simulink model "F550_Openloop"  (R2024a)
settings: Solver=VariableStepAuto  StartTime=0.0  StopTime=100  FixedStep=0.001  RelTol=1e-3
undefined symbols (not defined in the file): r2d
settings Model: Creator=ADMIN  LastModifiedBy=CNU_UASG
settings DataIOCC: ExternalInput=getinputstruct(op_trim1)  InitialState=getstatestruct(op_trim1)
settings DebuggingCC: UnconnectedInputMsg=warning  UnconnectedOutputMsg=warning  UnconnectedLineMsg=warning
settings ModelReferenceCC: EnableRefExpFcnMdlSchedulingChecks=on
settings RTWCC: GPUComputeCapability=3.5  DLArmComputeVersion=19.05

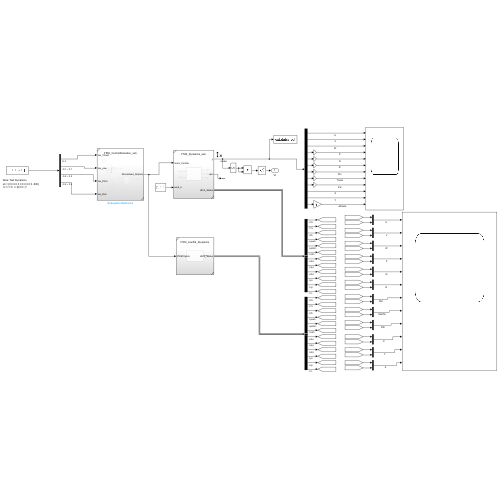
[thumbnail: Simulink's stored preview of the top-level diagram]
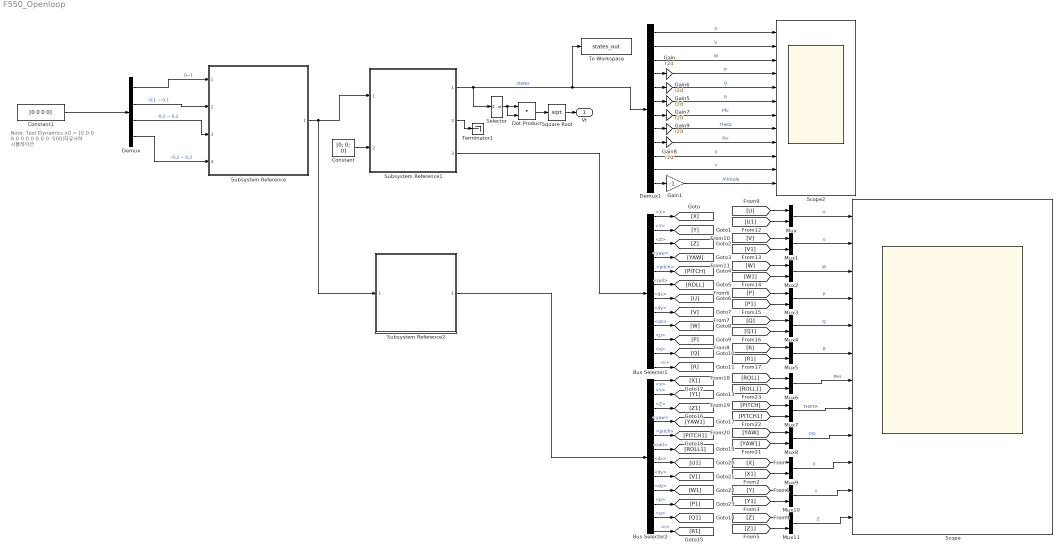
== system F550_Openloop ==
  note: Note: Test Dynamics
      | x0 = [0 0 0 0 0 0 0 0 0 0 0 -500]
      | 자유낙하 시뮬레이션
  Bus Selector1 : BusSelector  OutputSignals=X,Y,Z,yaw,pitch,roll,dx,dy,dz,p,q,r
  Bus Selector2 : BusSelector  OutputSignals=X,Y,Z,yaw,pitch,roll,dx,dy,dz,p,q,r
  Constant : Constant  Value=[0; 0; 0]
  Constant1 : Constant  Value=[0 0 0 0]
  Demux : Demux
  Demux1 : Demux  Outputs=12
  Dot Product : DotProduct  OutDataTypeStr=Inherit: Inherit via internal rule
  Gain{,5..9} (6 alike) : Gain  Gain=r2d
  Gain1 : Gain  Gain=-1
  Mux{,1..11} (12 alike) : Mux  Inputs=2
  Scope : Scope  NumInputPorts=12
  Scope2 : Scope  NumInputPorts=12
  Selector : Selector  InputPortWidth=12  IndexOptions=Index vector (dialog)  Indices=[1 2 3]  OutputSizes=1
  Square Root : Sqrt
  Subsystem Reference : Subsystem  ReferencedSubsystem=F550_ControlAllocation_sub
  Subsystem Reference1 : Subsystem  ReferencedSubsystem=F550_Dynamics_sub
  Subsystem Reference2 : Subsystem  ReferencedSubsystem=F550_LowFid_Dynamics
  Terminator1 : Terminator
  To Workspace : ToWorkspace  VariableName=states_out  SampleTime=-1
  Vt : Outport
  wires:
  Demux/4 -> Subsystem Reference/4  "-0.2 ~ 0.2"
  Demux/3 -> Subsystem Reference/3  "-0.2 ~ 0.2"
  Demux/2 -> Subsystem Reference/2  "-0.1 ~ 0.1"
  Demux/1 -> Subsystem Reference/1  "0~1"
  Selector/1 -> Dot Product/1, Dot Product/2
  Square Root/1 -> Vt/1
  Dot Product/1 -> Square Root/1
  Subsystem Reference1/1 -> Demux1/1, To Workspace/1, Selector/1  "states"
  Subsystem Reference1/3 -> Bus Selector1/1
  Constant/1 -> Subsystem Reference1/2
  Subsystem Reference/1 -> Subsystem Reference2/1, Subsystem Reference1/1
  Subsystem Reference1/2 -> Terminator1/1
  Gain5/1 -> Scope2/6  "R"
  Demux1/9 -> Gain8/1
  Demux1/7 -> Gain7/1
  Demux1/3 -> Scope2/3  "W"
  Demux1/1 -> Scope2/1  "U"
  Demux1/2 -> Scope2/2  "V"
  Demux1/4 -> Gain/1
  Gain8/1 -> Scope2/9  "Psi"
  Gain7/1 -> Scope2/7  "Phi"
  Demux1/8 -> Gain9/1
  Demux1/5 -> Gain6/1
  Gain/1 -> Scope2/4  "P"
  Gain6/1 -> Scope2/5  "Q"
  Gain9/1 -> Scope2/8  "Theta"
  Demux1/6 -> Gain5/1
  Demux1/10 -> Scope2/10  "X"
  Demux1/11 -> Scope2/11  "Y"
  Demux1/12 -> Gain1/1
  Gain1/1 -> Scope2/12  "Altitude"
  Constant1/1 -> Demux/1
  Subsystem Reference2/1 -> Bus Selector2/1
  [Y1] -> Mux10/2
  [V1] -> Mux1/2
  Mux7/1 -> Scope/8  "THETA"
  Bus Selector2/7 -> [U1]  "<dx>"
  [U] -> Mux/1
  Mux9/1 -> Scope/10  "X"
  Bus Selector1/1 -> [X]  "<X>"
  [Y] -> Mux10/1
  [X] -> Mux9/1
  [Z] -> Mux11/1
  [R1] -> Mux5/2
  Mux8/1 -> Scope/9  "PSI"
  Mux6/1 -> Scope/7  "PHI"
  Mux5/1 -> Scope/6  "R"
  Mux4/1 -> Scope/5  "Q"
  Mux1/1 -> Scope/2  "V"
  Bus Selector2/12 -> [R1]  "<r>"
  [W] -> Mux2/1
  [PITCH] -> Mux7/1
  [W1] -> Mux2/2
  Bus Selector1/11 -> [Q]  "<q>"
  [Z1] -> Mux11/2
  [R] -> Mux5/1
  Bus Selector2/3 -> [Z1]  "<Z>"
  [Q1] -> Mux4/2
  [YAW1] -> Mux8/2
  [P] -> Mux3/1
  [PITCH1] -> Mux7/2
  [V] -> Mux1/1
  [U1] -> Mux/2
  [P1] -> Mux3/2
  [Q] -> Mux4/1
  Bus Selector1/10 -> [P]  "<p>"
  Bus Selector2/10 -> [P1]  "<p>"
  [ROLL1] -> Mux6/2
  Mux10/1 -> Scope/11  "Y"
  [ROLL] -> Mux6/1
  Mux/1 -> Scope/1  "U"
  Bus Selector2/11 -> [Q1]  "<q>"
  Bus Selector2/4 -> [YAW1]  "<yaw>"
  Bus Selector1/12 -> [R]  "<r>"
  Bus Selector2/9 -> [W1]  "<dz>"
  [X1] -> Mux9/2
  Bus Selector2/6 -> [ROLL1]  "<roll>"
  Bus Selector2/2 -> [Y1]  "<Y>"
  Bus Selector2/1 -> [X1]  "<X>"
  Bus Selector1/7 -> [U]  "<dx>"
  [YAW] -> Mux8/1
  Bus Selector1/3 -> [Z]  "<Z>"
  Bus Selector2/5 -> [PITCH1]  "<pitch>"
  Bus Selector1/2 -> [Y]  "<Y>"
  Bus Selector1/4 -> [YAW]  "<yaw>"
  Mux3/1 -> Scope/4  "P"
  Bus Selector1/9 -> [W]  "<dz>"
  Bus Selector2/8 -> [V1]  "<dy>"
  Bus Selector1/5 -> [PITCH]  "<pitch>"
  Mux2/1 -> Scope/3  "W"
  Bus Selector1/8 -> [V]  "<dy>"
  Bus Selector1/6 -> [ROLL]  "<roll>"
  Mux11/1 -> Scope/12  "Z"
